simulink model "rrc_bw"  (Simulink 6.6)
settings: Solver=ode45  StartTime=0.0  StopTime=1  RelTol=1e-3
PreLoadFcn:
  | rrc_weights
  | filter_weights
StopFcn:
  | figure(15)
  | 
  | subplot(2,1,1)
  | plot(i_bb,'b');
  | xlabel('Samples');
  | ylabel('Amplitude');
  | legend('In Phase',1);
  | axis([0 10000 -1.5 1.5]);
  | 
  | subplot(2,1,2)
  | plot(q_bb,'k');
  | xlabel('Samples');
  | ylabel('Amplitude');
  | legend('Quadrature',1);
  | axis([0 10000 -1.5 1.5]);
  | 
  | doFFTplot(1/153.6e+3, i_if,'Modulated (I)',1,16);
  | doFFTplot(1/153.6e+3, q_if,'Modulated (Q)',1,17);
  | doFFTplot(1/153.6e+3, both_if,'Modulated (I + Q)',1,18);
libraries: dsparch4 x2, dspsigops x2
settings Model: Creator=lcrockett  LastModifiedBy=lcrockett

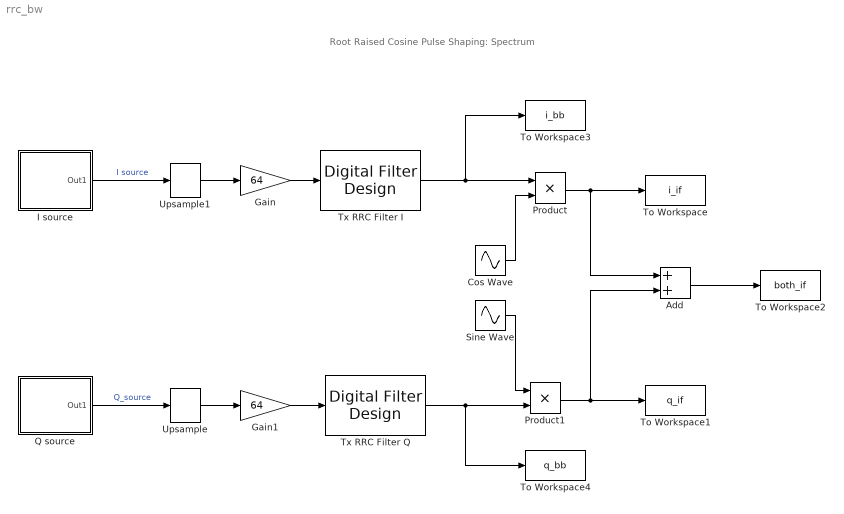
== system rrc_bw ==
  note: Root Raised Cosine Pulse Shaping: Spectrum
  Add : Sum  OutScaling=2^-10
  Cos Wave : Sin  Frequency=(38.4e+3)*2*pi  Phase=pi/2  SampleTime=1/153.6e+3
  Gain : Gain  Gain=64
  Gain1 : Gain  Gain=64
  I source : Subsystem
  Product : Product  RndMeth=Zero
  Product1 : Product  RndMeth=Zero
  Q source : Subsystem
  Sine Wave : Sin  Frequency=(38.4e+3)*2*pi  SampleTime=1/153.6e+3
  To Workspace : ToWorkspace  VariableName=i_if  SampleTime=-1  SaveFormat=Array
  To Workspace1 : ToWorkspace  VariableName=q_if  SampleTime=-1  SaveFormat=Array
  To Workspace2 : ToWorkspace  VariableName=both_if  SampleTime=-1  SaveFormat=Array
  To Workspace3 : ToWorkspace  VariableName=i_bb  SampleTime=-1  SaveFormat=Array
  To Workspace4 : ToWorkspace  VariableName=q_bb  SampleTime=-1  SaveFormat=Array
  Tx RRC Filter I : dsparch4/Digital Filter Design  SystemSampleTime=-1  mwdsp_browser_bugfix_var=off
  Tx RRC Filter Q : dsparch4/Digital Filter Design  SystemSampleTime=-1  mwdsp_browser_bugfix_var=off
  Upsample : dspsigops/Upsample  N=64  phase=0  ic=0  mode=Maintain input frame size
  Upsample1 : dspsigops/Upsample  N=64  phase=0  ic=0  mode=Maintain input frame size
  wires:
  Q source/1(Out1) -> Upsample/1  "Q_source"
  Tx RRC Filter I/1 -> Product/1, To Workspace3/1
  Tx RRC Filter Q/1 -> Product1/2, To Workspace4/1
  Product/1 -> Add/1, To Workspace/1
  Product1/1 -> Add/2, To Workspace1/1
  Upsample/1 -> Gain1/1
  I source/1(Out1) -> Upsample1/1  "I source"
  Upsample1/1 -> Gain/1
  Sine Wave/1 -> Product1/1
  Cos Wave/1 -> Product/2
  Gain/1 -> Tx RRC Filter I/1
  Gain1/1 -> Tx RRC Filter Q/1
  Add/1 -> To Workspace2/1

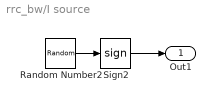
== system rrc_bw/I source ==
  Random Number2 : RandomNumber  Seed=777  SampleTime=1/2400
  Sign2 : Signum
  Out1 : Outport
  wires:
  Random Number2/1 -> Sign2/1
  Sign2/1 -> Out1/1

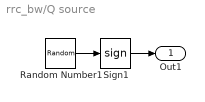
== system rrc_bw/Q source ==
  Random Number1 : RandomNumber  Seed=999  SampleTime=1/2400
  Sign1 : Signum
  Out1 : Outport
  wires:
  Random Number1/1 -> Sign1/1
  Sign1/1 -> Out1/1
